simulink model "T_Junction"  (R2021a)
settings: Solver=VariableStepAuto  StartTime=0.0  StopTime=10.0  RelTol=1e-3
libraries: EdgesLibrary x21, StreetLanesLibrary x18
settings Model: Creator=timyb  LastModifiedBy=timyb

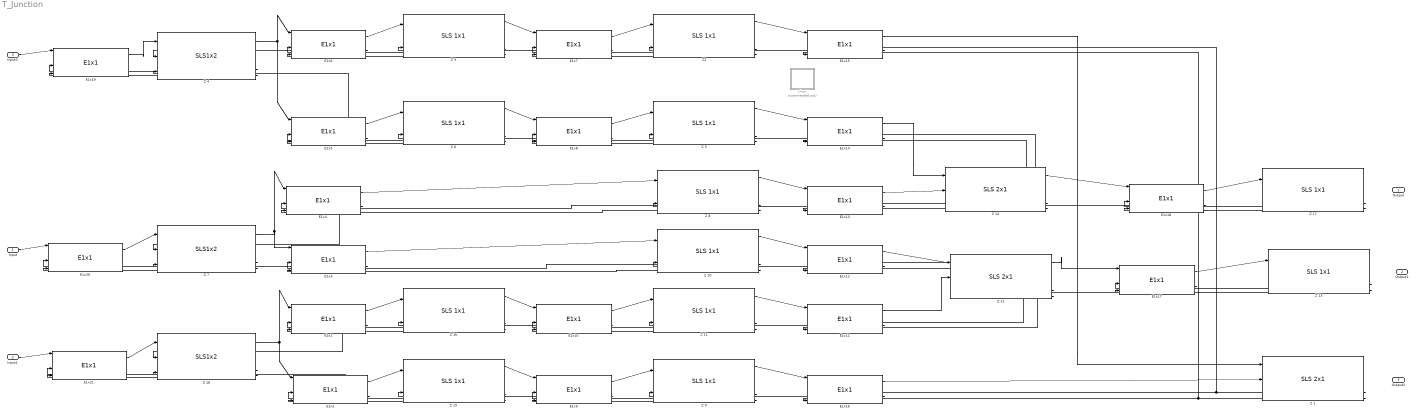
== system T_Junction ==
  Input : Inport
  Input1 : Inport  Port=2
  Input2 : Inport  Port=3
   Z {8..11,13,15..17} (8 alike) : StreetLanesLibrary/SLS 1x1  Kz=0  Tz=0
  " Z 3 " : StreetLanesLibrary/SLS 1x1  Kz=0  Tz=0
  Chart : Stateflow chart  Commented=on  TreatAsAtomicUnit=on
  E1x{1..21} (21 alike) : EdgesLibrary/E1x1
  "Z 1 " : StreetLanesLibrary/SLS 2x1  Kz=0  Tz=0
  Z 12 : StreetLanesLibrary/SLS 2x1  Kz=0  Tz=0
  Z 14 : StreetLanesLibrary/SLS 2x1  Kz=0  Tz=0
  Z 18 : StreetLanesLibrary/SLS1x2  Kz=0  Tz=0
  Z 4 : StreetLanesLibrary/SLS1x2  Kz=0  Tz=0
  "Z 5 " : StreetLanesLibrary/SLS 1x1  Kz=0  Tz=0
  "Z 6 " : StreetLanesLibrary/SLS 1x1  Kz=0  Tz=0
  Z 7 : StreetLanesLibrary/SLS1x2  Kz=0  Tz=0
  "Z2 " : StreetLanesLibrary/SLS 1x1  Kz=0  Tz=0
  Output : Outport
  Output1 : Outport  Port=2
  Output2 : Outport  Port=3
  wires:
  E1x6/2 -> Z 4/2
  Z 4/2 -> E1x6/1, E1x5/1
  E1x5/2 -> Z 4/3
  E1x5/1 -> "Z 6 "/1
  "Z 6 "/8 -> E1x5/4
  "Z 6 "/7 -> E1x5/3
  E1x6/1 -> " Z 3 "/1
  " Z 3 "/8 -> E1x6/4
  " Z 3 "/7 -> E1x6/3
  E1x7/2 -> " Z 3 "/2
  " Z 3 "/2 -> E1x7/1
  E1x8/2 -> "Z 6 "/2
  "Z 6 "/2 -> E1x8/1
  E1x7/1 -> "Z2 "/1
  "Z2 "/8 -> E1x7/4
  "Z2 "/7 -> E1x7/3
  E1x8/1 -> "Z 5 "/1
  "Z 5 "/8 -> E1x8/4
  "Z 5 "/7 -> E1x8/3
  Z 7/2 -> E1x4/1, E1x3/1
  E1x4/2 -> Z 7/2
  E1x3/2 -> Z 7/3
  " Z 10"/7 -> E1x3/3
  E1x3/1 -> " Z 10"/1
  " Z 10"/8 -> E1x3/4
  E1x4/1 -> " Z 8"/1
  " Z 8"/8 -> E1x4/4
  " Z 8"/7 -> E1x4/3
  E1x10/2 -> " Z 16"/2
  " Z 16"/2 -> E1x10/1
  E1x1/2 -> Z 18/2
  Z 18/2 -> E1x2/1, E1x1/1
  E1x2/2 -> Z 18/3
  E1x2/1 -> " Z 15"/1
  " Z 15"/8 -> E1x2/4
  " Z 15"/7 -> E1x2/3
  E1x1/1 -> " Z 16"/1
  " Z 16"/8 -> E1x1/4
  " Z 16"/7 -> E1x1/3
  E1x9/2 -> " Z 15"/2
  " Z 15"/2 -> E1x9/1
  E1x9/1 -> " Z 9"/1
  " Z 9"/8 -> E1x9/4
  " Z 9"/7 -> E1x9/3
  E1x10/1 -> " Z 11"/1
  " Z 11"/8 -> E1x10/4
  " Z 11"/7 -> E1x10/3
  E1x16/2 -> " Z 9"/2
  " Z 9"/2 -> E1x16/1
  E1x16/1 -> "Z 1 "/2
  E1x15/1 -> "Z 1 "/1
  "Z 1 "/8 -> E1x15/4, E1x16/4
  "Z 1 "/7 -> E1x16/3, E1x15/3
  E1x17/1 -> " Z 13"/1
  " Z 13"/8 -> E1x17/4
  " Z 13"/7 -> E1x17/3
  E1x17/2 -> Z 12/3
  Z 12/2 -> E1x17/1
  E1x11/1 -> Z 12/2
  Z 12/8 -> E1x12/4, E1x11/4
  Z 12/7 -> E1x12/3, E1x11/3
  E1x12/1 -> Z 12/1
  E1x11/2 -> " Z 11"/2
  " Z 11"/2 -> E1x11/1
  E1x12/2 -> " Z 10"/2
  " Z 10"/2 -> E1x12/1
  E1x13/2 -> " Z 8"/2
  " Z 8"/2 -> E1x13/1
  E1x14/2 -> "Z 5 "/2
  "Z 5 "/2 -> E1x14/1
  E1x13/1 -> Z 14/2
  E1x14/1 -> Z 14/1
  Z 14/8 -> E1x14/4, E1x13/4
  Z 14/7 -> E1x14/3, E1x13/3
  E1x18/2 -> Z 14/3
  Z 14/2 -> E1x18/1
  E1x18/1 -> " Z 17"/1
  " Z 17"/8 -> E1x18/4
  " Z 17"/7 -> E1x18/3
  E1x15/2 -> "Z2 "/2
  "Z2 "/2 -> E1x15/1
  Z 4/7 -> E1x19/3
  E1x19/1 -> Z 4/1
  Z 4/8 -> E1x19/4
  Input2/1 -> E1x19/1
  E1x20/1 -> Z 7/1
  Z 7/8 -> E1x20/4
  Z 7/7 -> E1x20/3
  Input/1 -> E1x20/1
  Input1/1 -> E1x21/1
  Z 18/7 -> E1x21/3
  Z 18/8 -> E1x21/4
  E1x21/1 -> Z 18/1

== stateflow chart T_Junction/Chart ==
  state Left
  state Right
  state Down
  Right -> Left
  Left -> Down
  Down -> Right
